simulink model "Constant4"  (R2017b)
settings: Solver=FixedStepDiscrete  StartTime=0.0  StopTime=19.8  FixedStep=0.200000  RelTol=1e-3
model workspace (MAT data in the model file):
  already_pp = 0
  input_struct.time = [0; 0.2; 0.4; 0.6; 0.8; 1; 1.2; 1.4; 1.6; 1.8; 2; 2.2; 2.4; 2.6; 2.8; 3; 3.2; 3.4; 3.6; 3.8; 4; 4.2; 4.4; 4.6; 4.8; 5; 5.2; 5.4; 5.6; 5.8; 6; 6.2; 6.4; 6.6; 6.8; 7; 7.2; 7.4; 7.6; 7.8; 8; 8.2; 8.4; 8.6; 8.8; 9; 9.2; 9.4; 9.6; 9.8; 10; 10.2; 10.4; 10.6; 10.8; 11; 11.2; 11.4; 11.6; 11.8; 12; 12.2; 12.4; 12.6; 12.8; 13; 13.2; 13.4; 13.6; 13.8; 14; 14.2; 14.4; 14.6; 14.8; 15; 15.2; 15.4; 15.6; 15.8; 16; 16.2; 16.4; 16.6; 16.8; 17; 17.2; 17.4; 17.6; 17.8; 18; 18.2; 18.4; 18.6; 18.8; 19; 19.2; 19.4; 19.6; 19.8]
  input_struct.signals.name = 'In5'
  input_struct.signals.values = [0; 1; 0; 0; 0; 1; 1; 1; 1; 0; 1; 0; 1; 1; 1; 0; 0; 1; 1; 1; 1; 1; 1; 1; 0; 1; 0; 0; 1; 0; 0; 1; 0; 0; 0; 0; 0; 1; 0; 0; 0; 0; 1; 0; 1; 1; 1; 1; 0; 0; 1; 0; 1; 1; 1; 0; 1; 0; 0; 0; 1; 1; 1; 1; 0; 1; 0; 1; 1; 1; 1; 1; 0; 0; 1; 0; 0; 0; 0; 1; 1; 1; 0; 1; 1; 1; 1; 0; 1; 0; 1; 1; 1; 0; 1; 0; 0; 1; 1; 0]
  input_struct.signals.dimensions = 1
undefined symbols (not defined in the file): Detector_DelayedFixedDurationResetFalse, pp_lib
settings Model: Creator=hbourbou  LastModifiedBy=hbourbou
settings DataIOCC: ExternalInput=input_struct  LoadExternalInput=on  SaveFormat=Structure  SaveState=on
settings OptimizationCC: LifeSpan=inf
settings DebuggingCC: AlgebraicLoopMsg=error  ArtificialAlgebraicLoopMsg=error  SFExecutionAtInitializationDiag=none
settings HardwareCC: ProdBitPerSizeT=32  ProdBitPerPtrDiffT=32  ProdWordSize=32  ProdHWDeviceType=Specified
settings CodeAppCC: StateflowObjectComments=on
settings GRTTargetCC: ExtMode=on

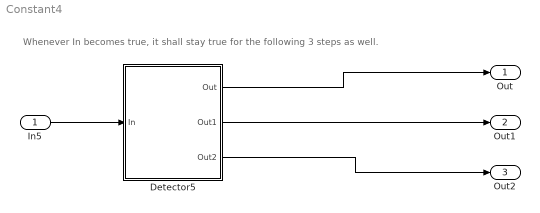
== system Constant4 ==
  note: Whenever In becomes true, it shall stay true for the following 3 steps as well.
  In5 : Inport  OutDataTypeStr=boolean  PortDimensions=1
  Detector5 : Subsystem  AncestorBlock=pp_lib/Detector_DelayedFixedDurationResetFalse  TreatAsAtomicUnit=on  mask(CoCoSim Detector Delayed Fixed Duration Reset False){in_hold=1, delay=2, out_hold=3}
      mask prompts: in_hold "Time steps for input detection"; delay "Time steps for delay (optional)"; out_hold "Time steps for output duration"
      mask Help: helpview(fullfile(docroot,'toolbox','sldv','sldv.map'),'detector')
      mask Display:
      | color('gray');
      |  plot([0.15 0.2 0.2 2.800000e-01],[ 0.7 0.7 8.500000e-01 8.500000e-01]);
      |  plot([3.100000e-01 3.800000e-01],[ 8.500000e-01 8.500000e-01]);
      |  plot([4.100000e-01 4.800000e-01],[ 8.500000e-01 8.500000e-01]);
      |  plot([5.100000e-01 5.800000e-01],[ 8.500000e-01 8.500000e-01]);
      |  plot([5.800000e-01 5.800000e-01],[0.7 0.75]);
      |  plot([5.800000e-01 5.800000e-01],[0.8 8.500000e-01]);
      |  plot([5.800000e-01 6.200000e-01],[ 7.000000e-01 7.000000e-01]);
      |  plot([6.500000e-01 0.75],[ 7.000000e-01 7.000000e-01]);
      |  color('black');
      |  plot([0.15 4.200000e-01 4.200000e-01 6.500000e-01 6.500000e-01 0.75], [3.300000e-01, 3.300000e-01 4.800000e-01 4.800000e-01 3.300000e-01 3.300000e-01]);
  Out : Outport  OutDataTypeStr=uint16
  Out1 : Outport  Port=2  OutDataTypeStr=uint16
  Out2 : Outport  Port=3  OutDataTypeStr=uint16
  wires:
  In5/1 -> Detector5/1(In)
  Detector5/3(Out2) -> Out2/1
  Detector5/1(Out) -> Out/1
  Detector5/2(Out1) -> Out1/1

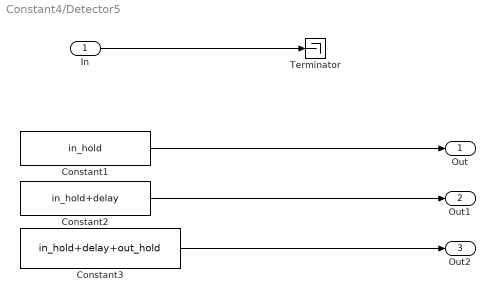
== system Constant4/Detector5 ==
  In : Inport  OutDataTypeStr=boolean  PortDimensions=1
  Constant1 : Constant  Value=in_hold  OutDataTypeStr=uint16
  Constant2 : Constant  Value=in_hold+delay  OutDataTypeStr=uint16
  Constant3 : Constant  Value=in_hold+delay+out_hold  OutDataTypeStr=uint16
  Terminator : Terminator
  Out : Outport  OutDataTypeStr=uint16
  Out1 : Outport  Port=2  OutDataTypeStr=uint16
  Out2 : Outport  Port=3  OutDataTypeStr=uint16
  wires:
  Constant3/1 -> Out2/1
  Constant2/1 -> Out1/1
  Constant1/1 -> Out/1
  In/1 -> Terminator/1
